simulink model "Bodies_6_Scissor_2_Stage"  (R2022b)
settings: Solver=ode15s  StartTime=0.0  StopTime=10.0  MaxStep=1e-2  RelTol=1e-3  AbsTol=1e-4  EnableMultiTasking=on
PostLoadFcn:
  | warning off Simulink:Engine:UsingDefaultMaxStepSize
  | warning off Simulink:Engine:InvActionDuringCallback
  | warning off sm:compiler:topologyAnalysis:DanglingBlock
  | warning off Simulink:Engine:LineWithoutDst
  | warning off Simulink:Engine:LineWithoutSrc
values from neighbouring files (symbols this model uses):
  rad = 5    [Plot_Extr_Data_Ring_withBoxFillet_forSlide.m]    (also in Plot_Link_Extr_Data_forSlide.m)
undefined symbols (not defined in the file or in its folder): SCL_Par, X, Y, Z
libraries: sm_lib x46, sm_scissor_lift_lib x12, nesl_utility x1
(part 2 of 2)

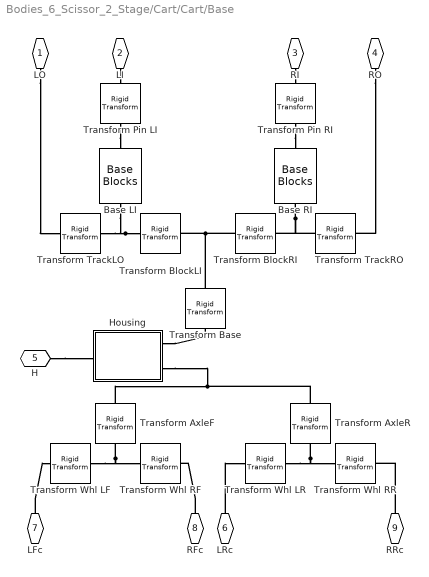
== system Bodies_6_Scissor_2_Stage/Cart/Cart/Base ==
  Base LI : sm_scissor_lift_lib/Base Blocks  block_length=SCL_Par.Base_Block.Length  block_width=SCL_Par.Base_Block.Width  block_height=SCL_Par.Base_Block.Height  shaft_radius=SCL_Par.Roller.Shaft_Radius  shaft_length=SCL_Par.Roller.Shaft_Length  material_density=SCL_Par.Base_Block.Density  material_color=SCL_Par.Base_Block.Color  material_opacity=SCL_Par.Base_Block.Opacity
  Base RI : sm_scissor_lift_lib/Base Blocks  block_length=SCL_Par.Base_Block.Length  block_width=SCL_Par.Base_Block.Width  block_height=SCL_Par.Base_Block.Height  shaft_radius=SCL_Par.Roller.Shaft_Radius  shaft_length=SCL_Par.Roller.Shaft_Length  material_density=SCL_Par.Base_Block.Density  material_color=SCL_Par.Base_Block.Color  material_opacity=SCL_Par.Base_Block.Opacity
  Housing : Subsystem
      mask Display: image('Block_IMAGE.jpg');
  Transform AxleF : sm_lib/Frames and Transforms/Rigid Transform  TranslationMethod=Cartesian  TranslationStandardOffset=0  TranslationLengthUnit=cm  TranslationStandardAxis=+Z  TranslationCartesianOffset=[SCL_Par.Cart.Axle.Wheelbase/2 0 -SCL_Par.Cart.Axle.Tire.Radius]  TranslationROffset=0  TranslationROffsetUnits=m  TranslationZOffset=0  TranslationZOffsetUnits=m  TranslationThetaOffset=0  TranslationThetaOffsetUnits=deg  RotationMethod=StandardAxis  RotationAngleUnits=deg  RotationStandardAxis=-X  RotationAngle=90  RotationArbitraryAxis=[0 0 1]  FollAlignAxisA=+X  BaseAlignAxisA=+Y  FollAlignAxisB=+Y  BaseAlignAxisB=+Z  RotationSequenceAxes=FollowerAxes  RotationSequence=XYX  RotationSequenceAngles=[0 0 0]  RotationSequenceAnglesUnits=deg  RotationMatrix=[1 0 0; 0 1 0; 0 0 1]  Quaternion=[1 0 0 0]
  Transform AxleR : sm_lib/Frames and Transforms/Rigid Transform  TranslationMethod=Cartesian  TranslationStandardOffset=0  TranslationLengthUnit=cm  TranslationStandardAxis=+Y  TranslationCartesianOffset=[-SCL_Par.Cart.Axle.Wheelbase/2 0 -SCL_Par.Cart.Axle.Tire.Radius]  TranslationROffset=0  TranslationROffsetUnits=m  TranslationZOffset=0  TranslationZOffsetUnits=m  TranslationThetaOffset=0  TranslationThetaOffsetUnits=deg  RotationMethod=StandardAxis  RotationAngleUnits=deg  RotationStandardAxis=-X  RotationAngle=90  RotationArbitraryAxis=[0 0 1]  FollAlignAxisA=+X  BaseAlignAxisA=+Y  FollAlignAxisB=+Y  BaseAlignAxisB=+Z  RotationSequenceAxes=FollowerAxes  RotationSequence=XYX  RotationSequenceAngles=[0 0 0]  RotationSequenceAnglesUnits=deg  RotationMatrix=[1 0 0; 0 1 0; 0 0 1]  Quaternion=[1 0 0 0]
  Transform Base : sm_lib/Frames and Transforms/Rigid Transform  TranslationMethod=Cartesian  TranslationStandardOffset=0  TranslationLengthUnit=cm  TranslationStandardAxis=+Y  TranslationCartesianOffset=[SCL_Par.Cart.Platform.Length/2-20 0 0]  TranslationROffset=0  TranslationROffsetUnits=m  TranslationZOffset=0  TranslationZOffsetUnits=m  TranslationThetaOffset=0  TranslationThetaOffsetUnits=deg  RotationMethod=StandardAxis  RotationAngleUnits=deg  RotationStandardAxis=+X  RotationAngle=90  RotationArbitraryAxis=[0 0 1]  FollAlignAxisA=+X  BaseAlignAxisA=+Y  FollAlignAxisB=+Y  BaseAlignAxisB=+Z  RotationSequenceAxes=FollowerAxes  RotationSequence=XYX  RotationSequenceAngles=[0 0 0]  RotationSequenceAnglesUnits=deg  RotationMatrix=[1 0 0; 0 1 0; 0 0 1]  Quaternion=[1 0 0 0]
  Transform BlockLI : sm_lib/Frames and Transforms/Rigid Transform  TranslationMethod=StandardAxis  TranslationStandardOffset=-SCL_Par.Link_Sep.Outer_Outer/2+SCL_Par.Link_Sep.Outer_Inner  TranslationLengthUnit=cm  TranslationStandardAxis=+Z  TranslationCartesianOffset=[0 0 0]  TranslationROffset=0  TranslationROffsetUnits=m  TranslationZOffset=0  TranslationZOffsetUnits=m  TranslationThetaOffset=0  TranslationThetaOffsetUnits=deg  RotationMethod=None  RotationAngleUnits=deg  RotationStandardAxis=+X  RotationAngle=90  RotationArbitraryAxis=[0 0 1]  FollAlignAxisA=+X  BaseAlignAxisA=+Y  FollAlignAxisB=+Y  BaseAlignAxisB=+Z  RotationSequenceAxes=FollowerAxes  RotationSequence=XYX  RotationSequenceAngles=[0 0 0]  RotationSequenceAnglesUnits=deg  RotationMatrix=[1 0 0; 0 1 0; 0 0 1]  Quaternion=[1 0 0 0]
  Transform BlockRI : sm_lib/Frames and Transforms/Rigid Transform  TranslationMethod=StandardAxis  TranslationStandardOffset=-SCL_Par.Link_Sep.Outer_Outer/2+SCL_Par.Link_Sep.Outer_Inner  TranslationLengthUnit=cm  TranslationStandardAxis=+Z  TranslationCartesianOffset=[0 0 0]  TranslationROffset=0  TranslationROffsetUnits=m  TranslationZOffset=0  TranslationZOffsetUnits=m  TranslationThetaOffset=0  TranslationThetaOffsetUnits=deg  RotationMethod=None  RotationAngleUnits=deg  RotationStandardAxis=+X  RotationAngle=90  RotationArbitraryAxis=[0 0 1]  FollAlignAxisA=+X  BaseAlignAxisA=+Y  FollAlignAxisB=+Y  BaseAlignAxisB=+Z  RotationSequenceAxes=FollowerAxes  RotationSequence=XYX  RotationSequenceAngles=[0 0 0]  RotationSequenceAnglesUnits=deg  RotationMatrix=[1 0 0; 0 1 0; 0 0 1]  Quaternion=[1 0 0 0]
  Transform Pin LI : sm_lib/Frames and Transforms/Rigid Transform  TranslationMethod=None  TranslationStandardOffset=0  TranslationLengthUnit=m  TranslationStandardAxis=+Z  TranslationCartesianOffset=[0 0 0]  TranslationROffset=0  TranslationROffsetUnits=m  TranslationZOffset=0  TranslationZOffsetUnits=m  TranslationThetaOffset=0  TranslationThetaOffsetUnits=deg  RotationMethod=StandardAxis  RotationAngleUnits=deg  RotationStandardAxis=+Z  RotationAngle=180  RotationArbitraryAxis=[0 0 1]  FollAlignAxisA=+X  BaseAlignAxisA=+Y  FollAlignAxisB=+Y  BaseAlignAxisB=+Z  RotationSequenceAxes=FollowerAxes  RotationSequence=XYX  RotationSequenceAngles=[0 0 0]  RotationSequenceAnglesUnits=deg  RotationMatrix=[1 0 0; 0 1 0; 0 0 1]  Quaternion=[1 0 0 0]
  Transform Pin RI : sm_lib/Frames and Transforms/Rigid Transform  TranslationMethod=None  TranslationStandardOffset=0  TranslationLengthUnit=m  TranslationStandardAxis=+Z  TranslationCartesianOffset=[0 0 0]  TranslationROffset=0  TranslationROffsetUnits=m  TranslationZOffset=0  TranslationZOffsetUnits=m  TranslationThetaOffset=0  TranslationThetaOffsetUnits=deg  RotationMethod=StandardAxis  RotationAngleUnits=deg  RotationStandardAxis=+Z  RotationAngle=180  RotationArbitraryAxis=[0 0 1]  FollAlignAxisA=+X  BaseAlignAxisA=+Y  FollAlignAxisB=+Y  BaseAlignAxisB=+Z  RotationSequenceAxes=FollowerAxes  RotationSequence=XYX  RotationSequenceAngles=[0 0 0]  RotationSequenceAnglesUnits=deg  RotationMatrix=[1 0 0; 0 1 0; 0 0 1]  Quaternion=[1 0 0 0]
  Transform TrackLO : sm_lib/Frames and Transforms/Rigid Transform  TranslationMethod=Cartesian  TranslationStandardOffset=0  TranslationLengthUnit=cm  TranslationStandardAxis=-Z  TranslationCartesianOffset=[0 SCL_Par.Roller.Roller_Radius -SCL_Par.Link_Sep.Outer_Inner]  TranslationROffset=0  TranslationROffsetUnits=m  TranslationZOffset=0  TranslationZOffsetUnits=m  TranslationThetaOffset=0  TranslationThetaOffsetUnits=deg  RotationMethod=StandardAxis  RotationAngleUnits=deg  RotationStandardAxis=+Y  RotationAngle=90  RotationArbitraryAxis=[0 0 1]  FollAlignAxisA=+X  BaseAlignAxisA=+Y  FollAlignAxisB=+Y  BaseAlignAxisB=+Z  RotationSequenceAxes=FollowerAxes  RotationSequence=XYX  RotationSequenceAngles=[0 0 0]  RotationSequenceAnglesUnits=deg  RotationMatrix=[1 0 0; 0 1 0; 0 0 1]  Quaternion=[1 0 0 0]
  Transform TrackRO : sm_lib/Frames and Transforms/Rigid Transform  TranslationMethod=Cartesian  TranslationStandardOffset=0  TranslationLengthUnit=cm  TranslationStandardAxis=+Z  TranslationCartesianOffset=[0 SCL_Par.Roller.Roller_Radius SCL_Par.Link_Sep.Outer_Inner]  TranslationROffset=0  TranslationROffsetUnits=m  TranslationZOffset=0  TranslationZOffsetUnits=m  TranslationThetaOffset=0  TranslationThetaOffsetUnits=deg  RotationMethod=StandardAxis  RotationAngleUnits=deg  RotationStandardAxis=+Y  RotationAngle=90  RotationArbitraryAxis=[0 0 1]  FollAlignAxisA=+X  BaseAlignAxisA=+Y  FollAlignAxisB=+Y  BaseAlignAxisB=+Z  RotationSequenceAxes=FollowerAxes  RotationSequence=XYX  RotationSequenceAngles=[0 0 0]  RotationSequenceAnglesUnits=deg  RotationMatrix=[1 0 0; 0 1 0; 0 0 1]  Quaternion=[1 0 0 0]
  "Transform Whl LF " : sm_lib/Frames and Transforms/Rigid Transform  TranslationMethod=StandardAxis  TranslationStandardOffset=SCL_Par.Cart.Axle.Wheel_Distance/2  TranslationLengthUnit=cm  TranslationStandardAxis=+Z  TranslationCartesianOffset=[0 0 0]  TranslationROffset=0  TranslationROffsetUnits=m  TranslationZOffset=0  TranslationZOffsetUnits=m  TranslationThetaOffset=0  TranslationThetaOffsetUnits=deg  RotationMethod=None  RotationAngleUnits=deg  RotationStandardAxis=-X  RotationAngle=90  RotationArbitraryAxis=[0 0 1]  FollAlignAxisA=+X  BaseAlignAxisA=+Y  FollAlignAxisB=+Y  BaseAlignAxisB=+Z  RotationSequenceAxes=FollowerAxes  RotationSequence=XYX  RotationSequenceAngles=[0 0 0]  RotationSequenceAnglesUnits=deg  RotationMatrix=[1 0 0; 0 1 0; 0 0 1]  Quaternion=[1 0 0 0]
  Transform Whl LR : sm_lib/Frames and Transforms/Rigid Transform  TranslationMethod=StandardAxis  TranslationStandardOffset=SCL_Par.Cart.Axle.Wheel_Distance/2  TranslationLengthUnit=cm  TranslationStandardAxis=+Z  TranslationCartesianOffset=[0 0 0]  TranslationROffset=0  TranslationROffsetUnits=m  TranslationZOffset=0  TranslationZOffsetUnits=m  TranslationThetaOffset=0  TranslationThetaOffsetUnits=deg  RotationMethod=None  RotationAngleUnits=deg  RotationStandardAxis=-X  RotationAngle=90  RotationArbitraryAxis=[0 0 1]  FollAlignAxisA=+X  BaseAlignAxisA=+Y  FollAlignAxisB=+Y  BaseAlignAxisB=+Z  RotationSequenceAxes=FollowerAxes  RotationSequence=XYX  RotationSequenceAngles=[0 0 0]  RotationSequenceAnglesUnits=deg  RotationMatrix=[1 0 0; 0 1 0; 0 0 1]  Quaternion=[1 0 0 0]
  Transform Whl RF : sm_lib/Frames and Transforms/Rigid Transform  TranslationMethod=StandardAxis  TranslationStandardOffset=SCL_Par.Cart.Axle.Wheel_Distance/2  TranslationLengthUnit=cm  TranslationStandardAxis=+Z  TranslationCartesianOffset=[0 0 0]  TranslationROffset=0  TranslationROffsetUnits=m  TranslationZOffset=0  TranslationZOffsetUnits=m  TranslationThetaOffset=0  TranslationThetaOffsetUnits=deg  RotationMethod=None  RotationAngleUnits=deg  RotationStandardAxis=-X  RotationAngle=90  RotationArbitraryAxis=[0 0 1]  FollAlignAxisA=+X  BaseAlignAxisA=+Y  FollAlignAxisB=+Y  BaseAlignAxisB=+Z  RotationSequenceAxes=FollowerAxes  RotationSequence=XYX  RotationSequenceAngles=[0 0 0]  RotationSequenceAnglesUnits=deg  RotationMatrix=[1 0 0; 0 1 0; 0 0 1]  Quaternion=[1 0 0 0]
  Transform Whl RR : sm_lib/Frames and Transforms/Rigid Transform  TranslationMethod=StandardAxis  TranslationStandardOffset=SCL_Par.Cart.Axle.Wheel_Distance/2  TranslationLengthUnit=cm  TranslationStandardAxis=+Z  TranslationCartesianOffset=[0 0 0]  TranslationROffset=0  TranslationROffsetUnits=m  TranslationZOffset=0  TranslationZOffsetUnits=m  TranslationThetaOffset=0  TranslationThetaOffsetUnits=deg  RotationMethod=None  RotationAngleUnits=deg  RotationStandardAxis=-X  RotationAngle=90  RotationArbitraryAxis=[0 0 1]  FollAlignAxisA=+X  BaseAlignAxisA=+Y  FollAlignAxisB=+Y  BaseAlignAxisB=+Z  RotationSequenceAxes=FollowerAxes  RotationSequence=XYX  RotationSequenceAngles=[0 0 0]  RotationSequenceAnglesUnits=deg  RotationMatrix=[1 0 0; 0 1 0; 0 0 1]  Quaternion=[1 0 0 0]
  LO : PMIOPort  Side=Right
  LI : PMIOPort  Port=2  Side=Right
  RI : PMIOPort  Port=3  Side=Right
  RO : PMIOPort  Port=4  Side=Right
  H : PMIOPort  Port=5  Side=Left
  LRc : PMIOPort  Port=6  Side=Left
  LFc : PMIOPort  Port=7  Side=Left
  RFc : PMIOPort  Port=8  Side=Left
  RRc : PMIOPort  Port=9  Side=Left
  connections:
  Transform Pin LI/LConn1 -- Base LI/RConn1
  RI/RConn1 -- Transform Pin RI/RConn1
  H/RConn1 -- Housing/LConn1
  Housing/RConn1 -- Transform Base/LConn1
  Transform AxleR/LConn1 -- Housing/RConn2 -- Transform AxleF/LConn1
  Base RI/LConn1 -- Transform BlockRI/LConn1 -- Transform TrackRO/LConn1
  Transform BlockLI/RConn1 -- Transform TrackLO/LConn1 -- Base LI/LConn1
  Transform BlockRI/RConn1 -- Transform BlockLI/LConn1 -- Transform Base/RConn1
  Transform AxleR/RConn1 -- Transform Whl LR/LConn1 -- Transform Whl RR/RConn1
  Transform AxleF/RConn1 -- Transform Whl RF/RConn1 -- "Transform Whl LF "/LConn1
  RO/RConn1 -- Transform TrackRO/RConn1
  LO/RConn1 -- Transform TrackLO/RConn1
  LI/RConn1 -- Transform Pin LI/RConn1
  Transform Pin RI/LConn1 -- Base RI/RConn1
  LRc/RConn1 -- Transform Whl LR/RConn1
  RRc/RConn1 -- Transform Whl RR/LConn1
  RFc/RConn1 -- Transform Whl RF/LConn1
  LFc/RConn1 -- "Transform Whl LF "/RConn1

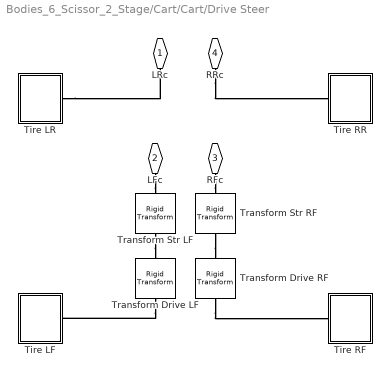
== system Bodies_6_Scissor_2_Stage/Cart/Cart/Drive Steer ==
  Tire LF : Subsystem  mask(Tire){Rt=SCL_Par.Cart.Axle.Tire.Radius, Tt=SCL_Par.Cart.Axle.Tire.Thickness, Rr=SCL_Par.Cart.Axle.Rim.Radius, Tr=SCL_Par.Cart.Axle.Rim.Thickness, rho=SCL_Par.Cart.Axle.Tire.Density, clr=SCL_Par.Cart.Axle.Tire.Color}
      mask prompts: Rt "Tire radius (cm)"; Tt "Tire thickness (cm)"; Rr "Rim radius (cm)"; Tr "Rim thickness (cm)"; rho "Density (kg/m^3)"; clr "Color"
      mask init:
      | theta = [(0:1:359) 0]'*pi/180;
      | unit_circle = [cos(theta), sin(theta)];
      | tire_sec = [Rt * unit_circle; Rr * flipud(unit_circle)];
      mask DialogControl ParameterTabVar0 Prompt: Dimensions
      mask DialogControl ParameterTabVar01 Prompt: Material Properties
      mask Display: image(imread('Scissor_Lift_Wheel_IMAGE.jpg'));
  Tire LR : Subsystem  mask(Tire){Rt=SCL_Par.Cart.Axle.Tire.Radius, Tt=SCL_Par.Cart.Axle.Tire.Thickness, Rr=SCL_Par.Cart.Axle.Rim.Radius, Tr=SCL_Par.Cart.Axle.Rim.Thickness, rho=SCL_Par.Cart.Axle.Tire.Density, clr=SCL_Par.Cart.Axle.Tire.Color}
      mask prompts: Rt "Tire radius (cm)"; Tt "Tire thickness (cm)"; Rr "Rim radius (cm)"; Tr "Rim thickness (cm)"; rho "Density (kg/m^3)"; clr "Color"
      mask init:
      | theta = [(0:1:359) 0]'*pi/180;
      | unit_circle = [cos(theta), sin(theta)];
      | tire_sec = [Rt * unit_circle; Rr * flipud(unit_circle)];
      mask DialogControl ParameterTabVar0 Prompt: Dimensions
      mask DialogControl ParameterTabVar01 Prompt: Material Properties
      mask Display: image(imread('Scissor_Lift_Wheel_IMAGE.jpg'));
  Tire RF : Subsystem  mask(Tire){Rt=SCL_Par.Cart.Axle.Tire.Radius, Tt=SCL_Par.Cart.Axle.Tire.Thickness, Rr=SCL_Par.Cart.Axle.Rim.Radius, Tr=SCL_Par.Cart.Axle.Rim.Thickness, rho=SCL_Par.Cart.Axle.Tire.Density, clr=SCL_Par.Cart.Axle.Tire.Color}
      mask prompts: Rt "Tire radius (cm)"; Tt "Tire thickness (cm)"; Rr "Rim radius (cm)"; Tr "Rim thickness (cm)"; rho "Density (kg/m^3)"; clr "Color"
      mask init:
      | theta = [(0:1:359) 0]'*pi/180;
      | unit_circle = [cos(theta), sin(theta)];
      | tire_sec = [Rt * unit_circle; Rr * flipud(unit_circle)];
      mask DialogControl ParameterTabVar0 Prompt: Dimensions
      mask DialogControl ParameterTabVar01 Prompt: Material Properties
      mask Display: image(imread('Scissor_Lift_Wheel_IMAGE.jpg'));
  Tire RR : Subsystem  mask(Tire){Rt=SCL_Par.Cart.Axle.Tire.Radius, Tt=SCL_Par.Cart.Axle.Tire.Thickness, Rr=SCL_Par.Cart.Axle.Rim.Radius, Tr=SCL_Par.Cart.Axle.Rim.Thickness, rho=SCL_Par.Cart.Axle.Tire.Density, clr=SCL_Par.Cart.Axle.Tire.Color}
      mask prompts: Rt "Tire radius (cm)"; Tt "Tire thickness (cm)"; Rr "Rim radius (cm)"; Tr "Rim thickness (cm)"; rho "Density (kg/m^3)"; clr "Color"
      mask init:
      | theta = [(0:1:359) 0]'*pi/180;
      | unit_circle = [cos(theta), sin(theta)];
      | tire_sec = [Rt * unit_circle; Rr * flipud(unit_circle)];
      mask DialogControl ParameterTabVar0 Prompt: Dimensions
      mask DialogControl ParameterTabVar01 Prompt: Material Properties
      mask Display: image(imread('Scissor_Lift_Wheel_IMAGE.jpg'));
  Transform Drive LF : sm_lib/Frames and Transforms/Rigid Transform  TranslationMethod=None  TranslationStandardOffset=0  TranslationLengthUnit=m  TranslationStandardAxis=+Z  TranslationCartesianOffset=[0 0 0]  TranslationROffset=0  TranslationROffsetUnits=m  TranslationZOffset=0  TranslationZOffsetUnits=m  TranslationThetaOffset=0  TranslationThetaOffsetUnits=deg  RotationMethod=StandardAxis  RotationAngleUnits=deg  RotationStandardAxis=+X  RotationAngle=90.0  RotationArbitraryAxis=[0 0 1]  FollAlignAxisA=+X  BaseAlignAxisA=+Y  FollAlignAxisB=+Y  BaseAlignAxisB=+Z  RotationSequenceAxes=FollowerAxes  RotationSequence=XYX  RotationSequenceAngles=[0 0 0]  RotationSequenceAnglesUnits=deg  RotationMatrix=[1 0 0; 0 1 0; 0 0 1]  Quaternion=[1 0 0 0]
  Transform Drive RF : sm_lib/Frames and Transforms/Rigid Transform  TranslationMethod=None  TranslationStandardOffset=0  TranslationLengthUnit=m  TranslationStandardAxis=+Z  TranslationCartesianOffset=[0 0 0]  TranslationROffset=0  TranslationROffsetUnits=m  TranslationZOffset=0  TranslationZOffsetUnits=m  TranslationThetaOffset=0  TranslationThetaOffsetUnits=deg  RotationMethod=StandardAxis  RotationAngleUnits=deg  RotationStandardAxis=+X  RotationAngle=90.0  RotationArbitraryAxis=[0 0 1]  FollAlignAxisA=+X  BaseAlignAxisA=+Y  FollAlignAxisB=+Y  BaseAlignAxisB=+Z  RotationSequenceAxes=FollowerAxes  RotationSequence=XYX  RotationSequenceAngles=[0 0 0]  RotationSequenceAnglesUnits=deg  RotationMatrix=[1 0 0; 0 1 0; 0 0 1]  Quaternion=[1 0 0 0]
  Transform Str LF : sm_lib/Frames and Transforms/Rigid Transform  TranslationMethod=None  TranslationStandardOffset=0  TranslationLengthUnit=m  TranslationStandardAxis=+Z  TranslationCartesianOffset=[0 0 0]  TranslationROffset=0  TranslationROffsetUnits=m  TranslationZOffset=0  TranslationZOffsetUnits=m  TranslationThetaOffset=0  TranslationThetaOffsetUnits=deg  RotationMethod=StandardAxis  RotationAngleUnits=deg  RotationStandardAxis=+X  RotationAngle=90.0  RotationArbitraryAxis=[0 0 1]  FollAlignAxisA=+X  BaseAlignAxisA=+Y  FollAlignAxisB=+Y  BaseAlignAxisB=+Z  RotationSequenceAxes=FollowerAxes  RotationSequence=XYX  RotationSequenceAngles=[0 0 0]  RotationSequenceAnglesUnits=deg  RotationMatrix=[1 0 0; 0 1 0; 0 0 1]  Quaternion=[1 0 0 0]
  "Transform Str RF " : sm_lib/Frames and Transforms/Rigid Transform  TranslationMethod=None  TranslationStandardOffset=0  TranslationLengthUnit=m  TranslationStandardAxis=+Z  TranslationCartesianOffset=[0 0 0]  TranslationROffset=0  TranslationROffsetUnits=m  TranslationZOffset=0  TranslationZOffsetUnits=m  TranslationThetaOffset=0  TranslationThetaOffsetUnits=deg  RotationMethod=StandardAxis  RotationAngleUnits=deg  RotationStandardAxis=+X  RotationAngle=90.0  RotationArbitraryAxis=[0 0 1]  FollAlignAxisA=+X  BaseAlignAxisA=+Y  FollAlignAxisB=+Y  BaseAlignAxisB=+Z  RotationSequenceAxes=FollowerAxes  RotationSequence=XYX  RotationSequenceAngles=[0 0 0]  RotationSequenceAnglesUnits=deg  RotationMatrix=[1 0 0; 0 1 0; 0 0 1]  Quaternion=[1 0 0 0]
  LRc : PMIOPort  Side=Left
  LFc : PMIOPort  Port=2  Side=Left
  RFc : PMIOPort  Port=3  Side=Left
  RRc : PMIOPort  Port=4  Side=Left
  connections:
  RFc/RConn1 -- "Transform Str RF "/LConn1
  LFc/RConn1 -- Transform Str LF/LConn1
  "Transform Str RF "/RConn1 -- Transform Drive RF/RConn1
  Transform Str LF/RConn1 -- Transform Drive LF/RConn1
  Tire LR/LConn1 -- LRc/RConn1
  RRc/RConn1 -- Tire RR/LConn1
  Transform Drive LF/LConn1 -- Tire LF/LConn1
  Transform Drive RF/LConn1 -- Tire RF/LConn1

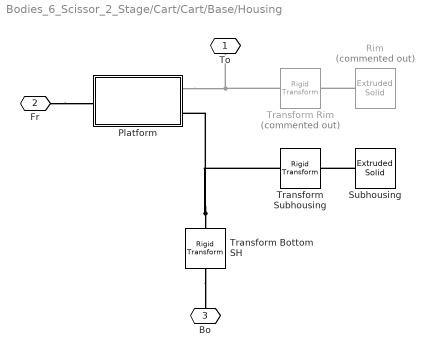
== system Bodies_6_Scissor_2_Stage/Cart/Cart/Base/Housing ==
  Platform : Subsystem  mask(Block){L=SCL_Par.Cart.Platform.Width, W=SCL_Par.Cart.Platform.Length, H=SCL_Par.Cart.Platform.Height, z_ori=Local +Z, rho=SCL_Par.Base_Block.Density, clr=SCL_Par.Base_Block.Color, opc=SCL_Par.Base_Block.Opacity}
      mask prompts: L "Length (cm):"; W "Width (cm):"; H "Height (cm):"; z_ori "Shaft orientation:"; rho "Shaft density (kg/m^3):"; clr "Link color:"; opc "Opacity:"
      mask help: Rectangular block. Ports are at the center of the faces normal to the local z-axis. Can be configured to have positive Z from B to F or from F to B.
      mask init:
      | if(z_ori == 2)
      |     z_ori = -1;
      | end
      mask TypeOptions z_ori: Local +Z | Local -Z
      mask DialogControl ParameterTabVar0 Prompt: Dimensions
      mask DialogControl ParameterTabVar01 Prompt: Material
      mask Display: image(imread('Block_IMAGE.jpg'));
  Rim : sm_lib/Body Elements/Extruded Solid  Commented=on  GraphicAmbientColor=[0.15 0.15 0.15 1.0]  BasedOnType=Density  CenterOfMass=[0 0 0]  CenterOfMassUnits=m  GraphicDiffuseColor=SCL_Par.Colors.Blue  ExportConvexHullGeometry=off  ExtrusionCrossSection=SCL_Par.Cart.Platform.Rim.Extrusion  ExtrusionCrossSectionUnits=cm  Density=1000  DensityUnits=kg/(m^3)  DoExposeReferenceFrame=on  GraphicEmissiveColor=[0.0 0.0 0.0 1.0]  ExportEntireGeometry=off  ExtrusionLength=SCL_Par.Cart.Platform.Rim.Depth  ExtrusionLengthUnits=cm  ExtrusionType=General  SerializedFrames=<Frames/>  MarkerShape=Sphere  MarkerSize=10  GraphicType=FromGeometry  InertiaType=CalculateFromGeometry  Mass=1  MassUnits=kg  MomentsOfInertia=[1 1 1]  MomentsOfInertiaUnits=kg*m^2  PolygonNumSides=3  GraphicOpacity=1.0  PolygonOuterRadius=1  PolygonOuterRadiusUnits=m  ProductsOfInertia=[0 0 0]  ProductsOfInertiaUnits=kg*m^2  GraphicShininess=75  GraphicSpecularColor=[0.5 0.5 0.5 1.0]  GraphicVisPropType=SimpleVisualProperties
  Subhousing : sm_lib/Body Elements/Extruded Solid  GraphicAmbientColor=[0.15 0.15 0.15 1.0]  BasedOnType=Density  CenterOfMass=[0 0 0]  CenterOfMassUnits=m  GraphicDiffuseColor=SCL_Par.Cart.Platform.Subhousing.Color  ExportConvexHullGeometry=off  ExtrusionCrossSection=SCL_Par.Cart.Platform.Subhousing.Extr  ExtrusionCrossSectionUnits=cm  Density=10  DensityUnits=kg/(m^3)  DoExposeReferenceFrame=on  GraphicEmissiveColor=[0.0 0.0 0.0 1.0]  ExportEntireGeometry=off  ExtrusionLength=SCL_Par.Cart.Platform.Width  ExtrusionLengthUnits=cm  ExtrusionType=General  SerializedFrames=<Frames/>  MarkerShape=Sphere  MarkerSize=10  GraphicType=FromGeometry  InertiaType=CalculateFromGeometry  Mass=1  MassUnits=kg  MomentsOfInertia=[1 1 1]  MomentsOfInertiaUnits=kg*m^2  PolygonNumSides=3  GraphicOpacity=1.0  PolygonOuterRadius=1  PolygonOuterRadiusUnits=m  ProductsOfInertia=[0 0 0]  ProductsOfInertiaUnits=kg*m^2  GraphicShininess=75  GraphicSpecularColor=[0.5 0.5 0.5 1.0]  GraphicVisPropType=SimpleVisualProperties
  Transform Bottom SH : sm_lib/Frames and Transforms/Rigid Transform  TranslationMethod=StandardAxis  TranslationStandardOffset=5  TranslationLengthUnit=cm  TranslationStandardAxis=-Z  TranslationCartesianOffset=[0 0 0]  TranslationROffset=0  TranslationROffsetUnits=m  TranslationZOffset=0  TranslationZOffsetUnits=m  TranslationThetaOffset=0  TranslationThetaOffsetUnits=deg  RotationMethod=None  RotationAngleUnits=deg  RotationStandardAxis=+X  RotationAngle=90.0  RotationArbitraryAxis=[0 0 1]  FollAlignAxisA=+X  BaseAlignAxisA=+Y  FollAlignAxisB=+Y  BaseAlignAxisB=+Z  RotationSequenceAxes=BaseAxes  RotationSequence=XZX  RotationSequenceAngles=[0 0 0]  RotationSequenceAnglesUnits=deg  RotationMatrix=[1 0 0; 0 1 0; 0 0 1]  Quaternion=[1 0 0 0]
  Transform Rim : sm_lib/Frames and Transforms/Rigid Transform  Commented=on  TranslationMethod=StandardAxis  TranslationStandardOffset=SCL_Par.Cart.Platform.Rim.Depth/2  TranslationLengthUnit=cm  TranslationStandardAxis=+Z  TranslationCartesianOffset=[0 0 0]  TranslationROffset=0  TranslationROffsetUnits=m  TranslationZOffset=0  TranslationZOffsetUnits=m  TranslationThetaOffset=0  TranslationThetaOffsetUnits=deg  RotationMethod=None  RotationAngleUnits=deg  RotationStandardAxis=+Z  RotationAngle=0.0  RotationArbitraryAxis=[0 0 1]  FollAlignAxisA=+X  BaseAlignAxisA=+Y  FollAlignAxisB=+Y  BaseAlignAxisB=+Z  RotationSequenceAxes=FollowerAxes  RotationSequence=XYX  RotationSequenceAngles=[0 0 0]  RotationSequenceAnglesUnits=deg  RotationMatrix=[1 0 0; 0 1 0; 0 0 1]  Quaternion=[1 0 0 0]
  Transform Subhousing : sm_lib/Frames and Transforms/Rigid Transform  TranslationMethod=None  TranslationStandardOffset=0  TranslationLengthUnit=m  TranslationStandardAxis=+Z  TranslationCartesianOffset=[0 0 0]  TranslationROffset=0  TranslationROffsetUnits=m  TranslationZOffset=0  TranslationZOffsetUnits=m  TranslationThetaOffset=0  TranslationThetaOffsetUnits=deg  RotationMethod=RotationSequence  RotationAngleUnits=deg  RotationStandardAxis=+X  RotationAngle=90.0  RotationArbitraryAxis=[0 0 1]  FollAlignAxisA=+X  BaseAlignAxisA=+Y  FollAlignAxisB=+Y  BaseAlignAxisB=+Z  RotationSequenceAxes=BaseAxes  RotationSequence=XZX  RotationSequenceAngles=[90 180 0]  RotationSequenceAnglesUnits=deg  RotationMatrix=[1 0 0; 0 1 0; 0 0 1]  Quaternion=[1 0 0 0]
  To : PMIOPort  Side=Right
  Fr : PMIOPort  Port=2  Side=Left
  Bo : PMIOPort  Port=3  Side=Right
  connections:
  Transform Bottom SH/LConn1 -- Platform/RConn2 -- Transform Subhousing/LConn1
  Transform Bottom SH/RConn1 -- Bo/RConn1
  Rim/RConn1 -- Transform Rim/RConn1
  Transform Rim/LConn1 -- To/RConn1 -- Platform/RConn1
  Fr/RConn1 -- Platform/LConn1
  Subhousing/RConn1 -- Transform Subhousing/RConn1

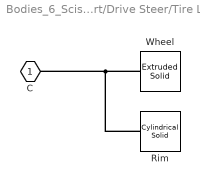
== system Bodies_6_Scissor_2_Stage/Cart/Cart/Drive Steer/Tire LF ==
  Rim : sm_lib/Body Elements/Cylindrical Solid  GraphicAmbientColor=[0.5 0.0 0.0 1.0]  BasedOnType=Density  CenterOfMass=[0 0 0]  CenterOfMassUnits=m  GraphicDiffuseColor=clr  CylinderLength=Tr  CylinderLengthUnits=cm  CylinderRadius=Rr  CylinderRadiusUnits=cm  Density=rho  DensityUnits=kg/(m^3)  DoExposeReferenceFrame=on  GraphicEmissiveColor=[0.0 0.0 0.0 1.0]  ExportEntireGeometry=off  SerializedFrames=<Frames/>  MarkerShape=Sphere  MarkerSize=10  GraphicType=FromGeometry  InertiaType=CalculateFromGeometry  Mass=1  MassUnits=kg  MomentsOfInertia=[1 1 1]  MomentsOfInertiaUnits=kg*m^2  GraphicOpacity=1.0  ProductsOfInertia=[0 0 0]  ProductsOfInertiaUnits=kg*m^2  GraphicShininess=75  GraphicSpecularColor=[0.5 0.5 0.5 1.0]  GraphicVisPropType=SimpleVisualProperties
  Wheel : sm_lib/Body Elements/Extruded Solid  GraphicAmbientColor=[0.5 0.0 0.0 1.0]  BasedOnType=Density  CenterOfMass=[0 0 0]  CenterOfMassUnits=m  GraphicDiffuseColor=clr  ExportConvexHullGeometry=off  ExtrusionCrossSection=tire_sec  ExtrusionCrossSectionUnits=cm  Density=rho  DensityUnits=kg/(m^3)  DoExposeReferenceFrame=on  GraphicEmissiveColor=[0.0 0.0 0.0 1.0]  ExportEntireGeometry=off  ExtrusionLength=Tt  ExtrusionLengthUnits=cm  ExtrusionType=General  SerializedFrames=<Frames/>  MarkerShape=Sphere  MarkerSize=10  GraphicType=FromGeometry  InertiaType=CalculateFromGeometry  Mass=1  MassUnits=kg  MomentsOfInertia=[1 1 1]  MomentsOfInertiaUnits=kg*m^2  PolygonNumSides=3  GraphicOpacity=1.0  PolygonOuterRadius=1  PolygonOuterRadiusUnits=m  ProductsOfInertia=[0 0 0]  ProductsOfInertiaUnits=kg*m^2  GraphicShininess=75  GraphicSpecularColor=[0.5 0.5 0.5 1.0]  GraphicVisPropType=SimpleVisualProperties
  C : PMIOPort  Side=Left
  connections:
  Wheel/RConn1 -- Rim/RConn1 -- C/RConn1

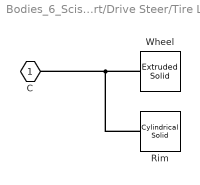
== system Bodies_6_Scissor_2_Stage/Cart/Cart/Drive Steer/Tire LR ==
  Rim : sm_lib/Body Elements/Cylindrical Solid  GraphicAmbientColor=[0.5 0.0 0.0 1.0]  BasedOnType=Density  CenterOfMass=[0 0 0]  CenterOfMassUnits=m  GraphicDiffuseColor=clr  CylinderLength=Tr  CylinderLengthUnits=cm  CylinderRadius=Rr  CylinderRadiusUnits=cm  Density=rho  DensityUnits=kg/(m^3)  DoExposeReferenceFrame=on  GraphicEmissiveColor=[0.0 0.0 0.0 1.0]  ExportEntireGeometry=off  SerializedFrames=<Frames/>  MarkerShape=Sphere  MarkerSize=10  GraphicType=FromGeometry  InertiaType=CalculateFromGeometry  Mass=1  MassUnits=kg  MomentsOfInertia=[1 1 1]  MomentsOfInertiaUnits=kg*m^2  GraphicOpacity=1.0  ProductsOfInertia=[0 0 0]  ProductsOfInertiaUnits=kg*m^2  GraphicShininess=75  GraphicSpecularColor=[0.5 0.5 0.5 1.0]  GraphicVisPropType=SimpleVisualProperties
  Wheel : sm_lib/Body Elements/Extruded Solid  GraphicAmbientColor=[0.5 0.0 0.0 1.0]  BasedOnType=Density  CenterOfMass=[0 0 0]  CenterOfMassUnits=m  GraphicDiffuseColor=clr  ExportConvexHullGeometry=off  ExtrusionCrossSection=tire_sec  ExtrusionCrossSectionUnits=cm  Density=rho  DensityUnits=kg/(m^3)  DoExposeReferenceFrame=on  GraphicEmissiveColor=[0.0 0.0 0.0 1.0]  ExportEntireGeometry=off  ExtrusionLength=Tt  ExtrusionLengthUnits=cm  ExtrusionType=General  SerializedFrames=<Frames/>  MarkerShape=Sphere  MarkerSize=10  GraphicType=FromGeometry  InertiaType=CalculateFromGeometry  Mass=1  MassUnits=kg  MomentsOfInertia=[1 1 1]  MomentsOfInertiaUnits=kg*m^2  PolygonNumSides=3  GraphicOpacity=1.0  PolygonOuterRadius=1  PolygonOuterRadiusUnits=m  ProductsOfInertia=[0 0 0]  ProductsOfInertiaUnits=kg*m^2  GraphicShininess=75  GraphicSpecularColor=[0.5 0.5 0.5 1.0]  GraphicVisPropType=SimpleVisualProperties
  C : PMIOPort  Side=Left
  connections:
  Wheel/RConn1 -- Rim/RConn1 -- C/RConn1

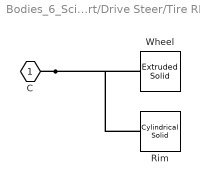
== system Bodies_6_Scissor_2_Stage/Cart/Cart/Drive Steer/Tire RF ==
  Rim : sm_lib/Body Elements/Cylindrical Solid  GraphicAmbientColor=[0.5 0.0 0.0 1.0]  BasedOnType=Density  CenterOfMass=[0 0 0]  CenterOfMassUnits=m  GraphicDiffuseColor=clr  CylinderLength=Tr  CylinderLengthUnits=cm  CylinderRadius=Rr  CylinderRadiusUnits=cm  Density=rho  DensityUnits=kg/(m^3)  DoExposeReferenceFrame=on  GraphicEmissiveColor=[0.0 0.0 0.0 1.0]  ExportEntireGeometry=off  SerializedFrames=<Frames/>  MarkerShape=Sphere  MarkerSize=10  GraphicType=FromGeometry  InertiaType=CalculateFromGeometry  Mass=1  MassUnits=kg  MomentsOfInertia=[1 1 1]  MomentsOfInertiaUnits=kg*m^2  GraphicOpacity=1.0  ProductsOfInertia=[0 0 0]  ProductsOfInertiaUnits=kg*m^2  GraphicShininess=75  GraphicSpecularColor=[0.5 0.5 0.5 1.0]  GraphicVisPropType=SimpleVisualProperties
  Wheel : sm_lib/Body Elements/Extruded Solid  GraphicAmbientColor=[0.5 0.0 0.0 1.0]  BasedOnType=Density  CenterOfMass=[0 0 0]  CenterOfMassUnits=m  GraphicDiffuseColor=clr  ExportConvexHullGeometry=off  ExtrusionCrossSection=tire_sec  ExtrusionCrossSectionUnits=cm  Density=rho  DensityUnits=kg/(m^3)  DoExposeReferenceFrame=on  GraphicEmissiveColor=[0.0 0.0 0.0 1.0]  ExportEntireGeometry=off  ExtrusionLength=Tt  ExtrusionLengthUnits=cm  ExtrusionType=General  SerializedFrames=<Frames/>  MarkerShape=Sphere  MarkerSize=10  GraphicType=FromGeometry  InertiaType=CalculateFromGeometry  Mass=1  MassUnits=kg  MomentsOfInertia=[1 1 1]  MomentsOfInertiaUnits=kg*m^2  PolygonNumSides=3  GraphicOpacity=1.0  PolygonOuterRadius=1  PolygonOuterRadiusUnits=m  ProductsOfInertia=[0 0 0]  ProductsOfInertiaUnits=kg*m^2  GraphicShininess=75  GraphicSpecularColor=[0.5 0.5 0.5 1.0]  GraphicVisPropType=SimpleVisualProperties
  C : PMIOPort  Side=Left
  connections:
  C/RConn1 -- Rim/RConn1 -- Wheel/RConn1

== system Bodies_6_Scissor_2_Stage/Cart/Cart/Drive Steer/Tire RR ==
  Rim : sm_lib/Body Elements/Cylindrical Solid  GraphicAmbientColor=[0.5 0.0 0.0 1.0]  BasedOnType=Density  CenterOfMass=[0 0 0]  CenterOfMassUnits=m  GraphicDiffuseColor=clr  CylinderLength=Tr  CylinderLengthUnits=cm  CylinderRadius=Rr  CylinderRadiusUnits=cm  Density=rho  DensityUnits=kg/(m^3)  DoExposeReferenceFrame=on  GraphicEmissiveColor=[0.0 0.0 0.0 1.0]  ExportEntireGeometry=off  SerializedFrames=<Frames/>  MarkerShape=Sphere  MarkerSize=10  GraphicType=FromGeometry  InertiaType=CalculateFromGeometry  Mass=1  MassUnits=kg  MomentsOfInertia=[1 1 1]  MomentsOfInertiaUnits=kg*m^2  GraphicOpacity=1.0  ProductsOfInertia=[0 0 0]  ProductsOfInertiaUnits=kg*m^2  GraphicShininess=75  GraphicSpecularColor=[0.5 0.5 0.5 1.0]  GraphicVisPropType=SimpleVisualProperties
  Wheel : sm_lib/Body Elements/Extruded Solid  GraphicAmbientColor=[0.5 0.0 0.0 1.0]  BasedOnType=Density  CenterOfMass=[0 0 0]  CenterOfMassUnits=m  GraphicDiffuseColor=clr  ExportConvexHullGeometry=off  ExtrusionCrossSection=tire_sec  ExtrusionCrossSectionUnits=cm  Density=rho  DensityUnits=kg/(m^3)  DoExposeReferenceFrame=on  GraphicEmissiveColor=[0.0 0.0 0.0 1.0]  ExportEntireGeometry=off  ExtrusionLength=Tt  ExtrusionLengthUnits=cm  ExtrusionType=General  SerializedFrames=<Frames/>  MarkerShape=Sphere  MarkerSize=10  GraphicType=FromGeometry  InertiaType=CalculateFromGeometry  Mass=1  MassUnits=kg  MomentsOfInertia=[1 1 1]  MomentsOfInertiaUnits=kg*m^2  PolygonNumSides=3  GraphicOpacity=1.0  PolygonOuterRadius=1  PolygonOuterRadiusUnits=m  ProductsOfInertia=[0 0 0]  ProductsOfInertiaUnits=kg*m^2  GraphicShininess=75  GraphicSpecularColor=[0.5 0.5 0.5 1.0]  GraphicVisPropType=SimpleVisualProperties
  C : PMIOPort  Side=Left
  connections:
  C/RConn1 -- Rim/RConn1 -- Wheel/RConn1

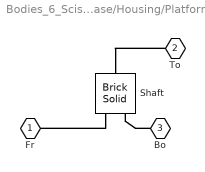
== system Bodies_6_Scissor_2_Stage/Cart/Cart/Base/Housing/Platform ==
  Shaft : sm_lib/Body Elements/Brick Solid  GraphicAmbientColor=[0.5 0.5 0.5]  BasedOnType=Density  BrickDimensions=[W L H]  BrickDimensionUnits=cm  CenterOfMass=[0 0 0]  CenterOfMassUnits=m  GraphicDiffuseColor=clr  Density=rho  DensityUnits=kg/m^3  DoExposeReferenceFrame=off  GraphicEmissiveColor=[0.1 0.1 0.1]  ExportEntireGeometry=off  SerializedFrames=<Frames><Frame><Id>Frame1</Id><Value><Name>Fr</Name><Origin><Source>GeometricFeature</Source><FeatureName>+x surface</FeatureName></Origin><PrimaryAxis><DefinedDirection>+Z</DefinedDirection><Source>ReferenceFrame</Source><SourceDirection>+Z</SourceDirection><FeatureName></FeatureName></PrimaryAxis><SecondaryAxis><DefinedDirection>+X</DefinedDirection><Source>ReferenceFrame</Source><SourceDirection>+X</SourceDirection><FeatureName></FeatureName></SecondaryAxis></Value></Frame><Frame><Id>Frame2</Id><Value><Name>To</Name><Origin><Source>GeometricFeature</Source><FeatureName>+z surface</FeatureName></Origin><PrimaryAxis><DefinedDirection>+Z</DefinedDirection><Source>ReferenceFrame</Source><SourceDirection>+Z</SourceDirection><FeatureName></FeatureName></PrimaryAxis><SecondaryAxis><DefinedDirection>+X</DefinedDirection><Source>ReferenceFrame</Source><SourceDirection>+X</SourceDirection><FeatureName></FeatureName></SecondaryAxis></Value></Frame><Frame><Id>Frame3</Id><Value><Name>Bo</Name><Origin><Source>GeometricFeature</Source><FeatureName>-z surface</FeatureName></Origin><PrimaryAxis><DefinedDirection>+Z</DefinedDirection><Source>ReferenceFrame</Source><SourceDirection>+Z</SourceDirection><FeatureName></FeatureName></PrimaryAxis><SecondaryAxis><DefinedDirection>+X</DefinedDirection><Source>ReferenceFrame</Source><SourceDirection>+X</SourceDirection><FeatureName></FeatureName></SecondaryAxis></Value></Frame></Frames>  MarkerShape=Sphere  MarkerSize=1  GraphicType=FromGeometry  InertiaType=CalculateFromGeometry  Mass=1  MassUnits=kg  MomentsOfInertia=[1 1 1]  MomentsOfInertiaUnits=kg*m^2  GraphicOpacity=opc  ProductsOfInertia=[0 0 0]  ProductsOfInertiaUnits=kg*m^2  GraphicShininess=24.0  GraphicSpecularColor=[0.2 0.2 0.2]  GraphicVisPropType=SimpleVisualProperties
  Fr : PMIOPort  Side=Left
  To : PMIOPort  Port=2  Side=Right
  Bo : PMIOPort  Port=3  Side=Right
  connections:
  Bo/RConn1 -- Shaft/LConn2
  To/RConn1 -- Shaft/RConn1
  Shaft/LConn1 -- Fr/RConn1
